simulink model "a1_walking"  (R2022b)
settings: Solver=VariableStepAuto  StartTime=0.0  StopTime=0.2  RelTol=1e-3
values from neighbouring files (symbols this model uses):
  m = 12    [MPC_Controller.m]    (also in QP_Controller.m; TASK1_rotating_mpc.m; TASK1_walking_backward_mpc.m; TASK1_walking_forward_mpc.m)
  N = 10    [MPC_Controller.m]
undefined symbols (not defined in the file or in its folder): X, Y, Z
libraries: sm_lib x188, nesl_utility x113
(part 2 of 5)

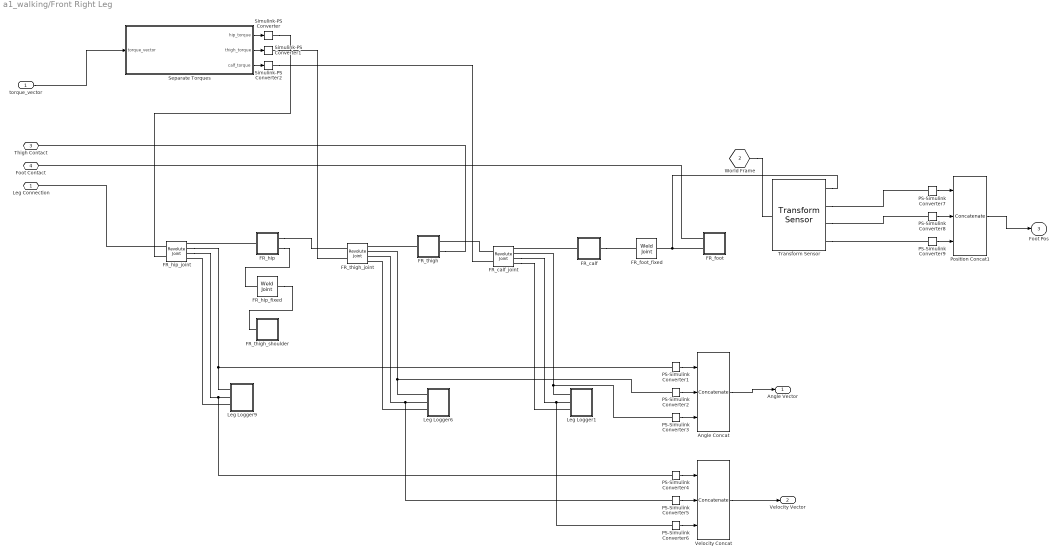
== system a1_walking/Front Right Leg ==
  torque_vector : Inport
  Angle Concat : Concatenate  NumInputs=3
  FR_calf : Subsystem
  FR_calf_joint : sm_lib/Joints/Revolute Joint  JointMode=Normal  SenseConstraintForce=off  SenseConstraintForceX=off  SenseConstraintForceY=off  SenseConstraintForceZ=off  SenseConstraintTorque=off  SenseConstraintTorqueX=off  SenseConstraintTorqueY=off  SenseConstraintTorqueZ=off  SenseTotalForce=off  SenseTotalForceX=off  SenseTotalForceY=off  SenseTotalForceZ=off  SenseTotalTorque=off  SenseTotalTorqueX=off  SenseTotalTorqueY=off  SenseTotalTorqueZ=off  CompositeWrenchDir=FollowerOnBase  CompositeWrenchFrame=BaseFrame  EquilibriumPosition=0  EquilibriumPositionUnits=deg  SpringStiffness=0  SpringStiffnessUnits=N*m/deg  DampingCoefficient=0.01  DampingCoefficientUnits=kg*m^2/(rad*s)  TorqueActuationMode=InputTorque  MotionActuationMode=ComputedMotion  SensePosition=on  SenseVelocity=on  SenseAcceleration=off  SenseTorqueForce=on  SenseLowerLimitTorqueForce=off  SenseUpperLimitTorqueForce=off  LowerLimitSpecify=on  LowerLimitBound=-2.69653369433  LowerLimitBoundUnits=rad  LowerLimitStiffness=1e4  LowerLimitStiffnessUnits=N*m/deg  LowerLimitDamping=10  LowerLimitDampingUnits=N*m/(deg/s)  LowerLimitTransitionRegionWidth=0.1  LowerLimitTransitionRegionWidthUnits=deg  UpperLimitSpecify=on  UpperLimitBound=-0.916297857297  UpperLimitBoundUnits=rad  UpperLimitStiffness=1e4  UpperLimitStiffnessUnits=N*m/deg  UpperLimitDamping=10  UpperLimitDampingUnits=N*m/(deg/s)  UpperLimitTransitionRegionWidth=0.1  UpperLimitTransitionRegionWidthUnits=deg  PositionTargetSpecify=on  PositionTargetPriority=High  PositionTargetValue=-2.5  PositionTargetValueUnits=rad  VelocityTargetSpecify=on  VelocityTargetPriority=High  VelocityTargetValue=0  VelocityTargetValueUnits=rad/s
  FR_foot : Subsystem
  FR_foot_fixed : sm_lib/Joints/Weld Joint  JointMode=Normal  SenseConstraintForce=off  SenseConstraintForceX=off  SenseConstraintForceY=off  SenseConstraintForceZ=off  SenseConstraintTorque=off  SenseConstraintTorqueX=off  SenseConstraintTorqueY=off  SenseConstraintTorqueZ=off  SenseTotalForce=off  SenseTotalForceX=off  SenseTotalForceY=off  SenseTotalForceZ=off  SenseTotalTorque=off  SenseTotalTorqueX=off  SenseTotalTorqueY=off  SenseTotalTorqueZ=off  CompositeWrenchDir=FollowerOnBase  CompositeWrenchFrame=BaseFrame
  FR_hip : Subsystem
  FR_hip_fixed : sm_lib/Joints/Weld Joint  JointMode=Normal  SenseConstraintForce=off  SenseConstraintForceX=off  SenseConstraintForceY=off  SenseConstraintForceZ=off  SenseConstraintTorque=off  SenseConstraintTorqueX=off  SenseConstraintTorqueY=off  SenseConstraintTorqueZ=off  SenseTotalForce=off  SenseTotalForceX=off  SenseTotalForceY=off  SenseTotalForceZ=off  SenseTotalTorque=off  SenseTotalTorqueX=off  SenseTotalTorqueY=off  SenseTotalTorqueZ=off  CompositeWrenchDir=FollowerOnBase  CompositeWrenchFrame=BaseFrame
  FR_hip_joint : sm_lib/Joints/Revolute Joint  JointMode=Normal  SenseConstraintForce=off  SenseConstraintForceX=off  SenseConstraintForceY=off  SenseConstraintForceZ=off  SenseConstraintTorque=off  SenseConstraintTorqueX=off  SenseConstraintTorqueY=off  SenseConstraintTorqueZ=off  SenseTotalForce=off  SenseTotalForceX=off  SenseTotalForceY=off  SenseTotalForceZ=off  SenseTotalTorque=off  SenseTotalTorqueX=off  SenseTotalTorqueY=off  SenseTotalTorqueZ=off  CompositeWrenchDir=FollowerOnBase  CompositeWrenchFrame=BaseFrame  EquilibriumPosition=0  EquilibriumPositionUnits=deg  SpringStiffness=0  SpringStiffnessUnits=N*m/deg  DampingCoefficient=0.01  DampingCoefficientUnits=kg*m^2/(rad*s)  TorqueActuationMode=InputTorque  MotionActuationMode=ComputedMotion  SensePosition=on  SenseVelocity=on  SenseAcceleration=off  SenseTorqueForce=on  SenseLowerLimitTorqueForce=off  SenseUpperLimitTorqueForce=off  LowerLimitSpecify=on  LowerLimitBound=-0.802851455917  LowerLimitBoundUnits=rad  LowerLimitStiffness=1e4  LowerLimitStiffnessUnits=N*m/deg  LowerLimitDamping=10  LowerLimitDampingUnits=N*m/(deg/s)  LowerLimitTransitionRegionWidth=0.1  LowerLimitTransitionRegionWidthUnits=deg  UpperLimitSpecify=on  UpperLimitBound=0.802851455917  UpperLimitBoundUnits=rad  UpperLimitStiffness=1e4  UpperLimitStiffnessUnits=N*m/deg  UpperLimitDamping=10  UpperLimitDampingUnits=N*m/(deg/s)  UpperLimitTransitionRegionWidth=0.1  UpperLimitTransitionRegionWidthUnits=deg  PositionTargetSpecify=on  PositionTargetPriority=High  PositionTargetValue=0  PositionTargetValueUnits=rad  VelocityTargetSpecify=on  VelocityTargetPriority=High  VelocityTargetValue=0  VelocityTargetValueUnits=deg/s
  FR_thigh : Subsystem
  FR_thigh_joint : sm_lib/Joints/Revolute Joint  JointMode=Normal  SenseConstraintForce=off  SenseConstraintForceX=off  SenseConstraintForceY=off  SenseConstraintForceZ=off  SenseConstraintTorque=off  SenseConstraintTorqueX=off  SenseConstraintTorqueY=off  SenseConstraintTorqueZ=off  SenseTotalForce=off  SenseTotalForceX=off  SenseTotalForceY=off  SenseTotalForceZ=off  SenseTotalTorque=off  SenseTotalTorqueX=off  SenseTotalTorqueY=off  SenseTotalTorqueZ=off  CompositeWrenchDir=FollowerOnBase  CompositeWrenchFrame=BaseFrame  EquilibriumPosition=0  EquilibriumPositionUnits=deg  SpringStiffness=0  SpringStiffnessUnits=N*m/deg  DampingCoefficient=0.01  DampingCoefficientUnits=kg*m^2/(rad*s)  TorqueActuationMode=InputTorque  MotionActuationMode=ComputedMotion  SensePosition=on  SenseVelocity=on  SenseAcceleration=off  SenseTorqueForce=on  SenseLowerLimitTorqueForce=off  SenseUpperLimitTorqueForce=off  LowerLimitSpecify=on  LowerLimitBound=-1.0471975512  LowerLimitBoundUnits=rad  LowerLimitStiffness=1e4  LowerLimitStiffnessUnits=N*m/deg  LowerLimitDamping=10  LowerLimitDampingUnits=N*m/(deg/s)  LowerLimitTransitionRegionWidth=0.1  LowerLimitTransitionRegionWidthUnits=deg  UpperLimitSpecify=on  UpperLimitBound=4.18879020479  UpperLimitBoundUnits=rad  UpperLimitStiffness=1e4  UpperLimitStiffnessUnits=N*m/deg  UpperLimitDamping=10  UpperLimitDampingUnits=N*m/(deg/s)  UpperLimitTransitionRegionWidth=0.1  UpperLimitTransitionRegionWidthUnits=deg  PositionTargetSpecify=on  PositionTargetPriority=High  PositionTargetValue=1  PositionTargetValueUnits=rad  VelocityTargetSpecify=on  VelocityTargetPriority=High  VelocityTargetValue=0  VelocityTargetValueUnits=deg/s
  FR_thigh_shoulder : Subsystem
  Leg Logger1 : Subsystem
  Leg Logger6 : Subsystem
  Leg Logger9 : Subsystem
  PS-Simulink Converter{1..9} (9 alike) : nesl_utility/PS-Simulink Converter  PhysicalDomain=network_engine_domain  SubClassName=ps_output  LeftPortType=input  RightPortType=output  PseudoPeriodic=off  Frequencies=[]  VectorFormat=inherit  Unit=inherit  AffineConversion=off
  Position Concat1 : Concatenate  NumInputs=3
  Separate Torques : MATLAB Function  TreatAsAtomicUnit=on
  Simulink-PS Converter : nesl_utility/Simulink-PS Converter  PhysicalDomain=network_engine_domain  SubClassName=ps_input  LeftPortType=input  RightPortType=output  PseudoPeriodic=off  Frequencies=[]  NoiseDistribution=none  NoiseParameters=[]  Unit=1  AffineConversion=off  FilteringAndDerivatives=provide  SimscapeFilterOrder=1  InputFilterTimeConstant=0.001  UdotUserProvided=0
  Simulink-PS Converter1 : nesl_utility/Simulink-PS Converter  PhysicalDomain=network_engine_domain  SubClassName=ps_input  LeftPortType=input  RightPortType=output  PseudoPeriodic=off  Frequencies=[]  NoiseDistribution=none  NoiseParameters=[]  Unit=1  AffineConversion=off  FilteringAndDerivatives=provide  SimscapeFilterOrder=1  InputFilterTimeConstant=0.001  UdotUserProvided=0
  Simulink-PS Converter2 : nesl_utility/Simulink-PS Converter  PhysicalDomain=network_engine_domain  SubClassName=ps_input  LeftPortType=input  RightPortType=output  PseudoPeriodic=off  Frequencies=[]  NoiseDistribution=none  NoiseParameters=[]  Unit=1  AffineConversion=off  FilteringAndDerivatives=provide  SimscapeFilterOrder=1  InputFilterTimeConstant=0.001  UdotUserProvided=0
  Transform Sensor : sm_lib/Frames and Transforms/Transform Sensor  MeasurementFrame=World  SenseAngle=off  SenseAxis=off  SenseQ=off  SenseR=off  SenseRotationSequence=off  RotationSequence=XYX  SenseOmegaX=off  SenseOmegaY=off  SenseOmegaZ=off  SenseQDot=off  SenseRDot=off  SenseAlphaX=off  SenseAlphaY=off  SenseAlphaZ=off  SenseQDDot=off  SenseRDDot=off  SenseX=on  SenseY=on  SenseZ=on  SenseRad=off  SenseAzim=off  SenseDist=off  SenseInc=off  SenseXDot=off  SenseYDot=off  SenseZDot=off  SenseRadDot=off  SenseAzimDot=off  SenseDistDot=off  SenseIncDot=off  SenseXDDot=off  SenseYDDot=off  SenseZDDot=off  SenseRadDDot=off  SenseAzimDDot=off  SenseDistDDot=off  SenseIncDDot=off
  Velocity Concat : Concatenate  NumInputs=3
  Leg Connection : PMIOPort  Side=Left
  World Frame : PMIOPort  Port=2  Side=Left
  Thigh Contact : PMIOPort  Port=3  Side=Left
  Foot Contact : PMIOPort  Port=4  Side=Left
  Angle Vector : Outport
  Velocity Vector : Outport  Port=2
  Foot Pos : Outport  Port=3
  wires:
  Separate Torques/2(thigh_torque) -> Simulink-PS Converter1/1
  Separate Torques/1(hip_torque) -> Simulink-PS Converter/1
  Separate Torques/3(calf_torque) -> Simulink-PS Converter2/1
  Velocity Concat/1 -> Velocity Vector/1
  PS-Simulink Converter4/1 -> Velocity Concat/1
  PS-Simulink Converter3/1 -> Angle Concat/3
  PS-Simulink Converter1/1 -> Angle Concat/1
  PS-Simulink Converter6/1 -> Velocity Concat/3
  PS-Simulink Converter5/1 -> Velocity Concat/2
  PS-Simulink Converter2/1 -> Angle Concat/2
  torque_vector/1 -> Separate Torques/1(torque_vector)
  Angle Concat/1 -> Angle Vector/1
  PS-Simulink Converter9/1 -> Position Concat1/3
  PS-Simulink Converter8/1 -> Position Concat1/2
  PS-Simulink Converter7/1 -> Position Concat1/1
  Position Concat1/1 -> Foot Pos/1
  connections:
  FR_calf_joint/RConn3 -- PS-Simulink Converter6/LConn1 -- Leg Logger1/LConn2
  Leg Logger6/LConn2 -- PS-Simulink Converter5/LConn1 -- FR_thigh_joint/RConn3
  Leg Logger6/LConn1 -- FR_thigh_joint/RConn2 -- PS-Simulink Converter2/LConn1
  FR_calf_joint/RConn4 -- Leg Logger1/LConn3
  FR_hip/RConn1 -- FR_thigh_joint/LConn1
  FR_thigh/LConn1 -- FR_thigh_joint/RConn1
  FR_hip_joint/RConn2 -- PS-Simulink Converter1/LConn1 -- Leg Logger9/LConn1
  Leg Logger9/LConn3 -- FR_hip_joint/RConn4
  FR_hip_fixed/RConn1 -- FR_thigh_shoulder/LConn1
  FR_calf_joint/LConn1 -- FR_thigh/RConn1
  Leg Logger6/LConn3 -- FR_thigh_joint/RConn4
  FR_hip/RConn2 -- FR_hip_fixed/LConn1
  FR_hip_joint/RConn3 -- PS-Simulink Converter4/LConn1 -- Leg Logger9/LConn2
  FR_thigh/RConn2 -- Thigh Contact/RConn1
  FR_hip_joint/LConn1 -- Leg Connection/RConn1
  Leg Logger1/LConn1 -- PS-Simulink Converter3/LConn1 -- FR_calf_joint/RConn2
  FR_calf/LConn1 -- FR_calf_joint/RConn1
  FR_calf/RConn1 -- FR_foot_fixed/LConn1
  FR_hip/LConn1 -- FR_hip_joint/RConn1
  FR_foot/LConn1 -- Foot Contact/RConn1
  FR_foot/LConn2 -- Transform Sensor/RConn1 -- FR_foot_fixed/RConn1
  Simulink-PS Converter1/RConn1 -- FR_thigh_joint/LConn2
  Simulink-PS Converter/RConn1 -- FR_hip_joint/LConn2
  Simulink-PS Converter2/RConn1 -- FR_calf_joint/LConn2
  Transform Sensor/RConn2 -- PS-Simulink Converter7/LConn1
  Transform Sensor/RConn3 -- PS-Simulink Converter8/LConn1
  Transform Sensor/RConn4 -- PS-Simulink Converter9/LConn1
  World Frame/RConn1 -- Transform Sensor/LConn1

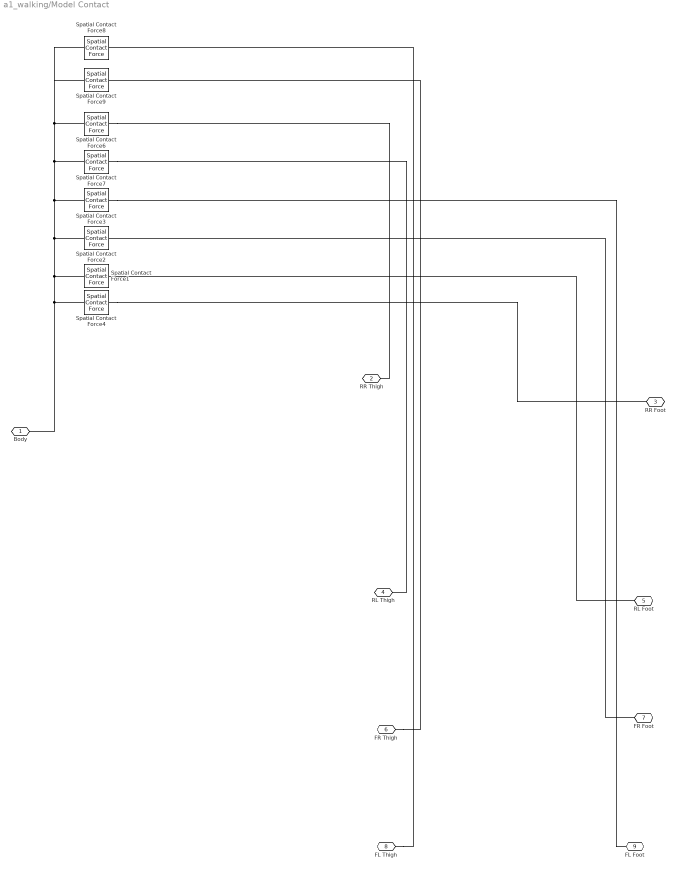
== system a1_walking/Model Contact ==
  Spatial Contact Force{1..4,6..9} (8 alike) : sm_lib/Forces and Torques/Spatial Contact Force  SenseContactBaseRotation=off  SenseContactBaseTranslation=off  CoefficientOfDynamicFriction=0.3  CoefficientOfStaticFriction=0.5  NormalDamping=1e3  NormalDampingUnits=N/(m/s)  SenseContactSignal=off  NormalStiffness=1e6  NormalStiffnessUnits=N/m  FrictionalCriticalVelocity=1e-3  FrictionalCriticalVelocityUnits=m/s  ZeroCrossDetectContactStartAndEnd=off  SenseContactFollowerRotation=off  SenseContactFollowerTranslation=off  FrictionType=SmoothStickSlip  SenseFrictionalForceMagnitude=off  SenseNormalForceMagnitude=off  NormalForceType=SmoothSpringDamper  SenseNormalVelocity=off  SenseSeparationDistance=off  SenseTangentialVelocity=off  NormalTransitionRegionWidth=1e-4  NormalTransitionRegionWidthUnits=m
  Body : PMIOPort  Side=Left
  RR Thigh : PMIOPort  Port=2  Side=Right
  RR Foot : PMIOPort  Port=3  Side=Right
  RL Thigh : PMIOPort  Port=4  Side=Right
  RL Foot : PMIOPort  Port=5  Side=Right
  FR Thigh : PMIOPort  Port=6  Side=Right
  FR Foot : PMIOPort  Port=7  Side=Right
  FL Thigh : PMIOPort  Port=8  Side=Right
  FL Foot : PMIOPort  Port=9  Side=Right
  connections:
  Spatial Contact Force3/RConn1 -- FL Foot/RConn1
  FL Thigh/RConn1 -- Spatial Contact Force8/RConn1
  Spatial Contact Force7/RConn1 -- RL Thigh/RConn1
  RL Foot/RConn1 -- Spatial Contact Force1/RConn1
  FR Thigh/RConn1 -- Spatial Contact Force9/RConn1
  Spatial Contact Force4/LConn1 -- Body/RConn1 -- Spatial Contact Force7/LConn1 -- Spatial Contact Force6/LConn1 -- Spatial Contact Force9/LConn1 -- Spatial Contact Force8/LConn1 -- Spatial Contact Force3/LConn1 -- Spatial Contact Force2/LConn1 -- Spatial Contact Force1/LConn1
  FR Foot/RConn1 -- Spatial Contact Force2/RConn1
  Spatial Contact Force6/RConn1 -- RR Thigh/RConn1
  Spatial Contact Force4/RConn1 -- RR Foot/RConn1

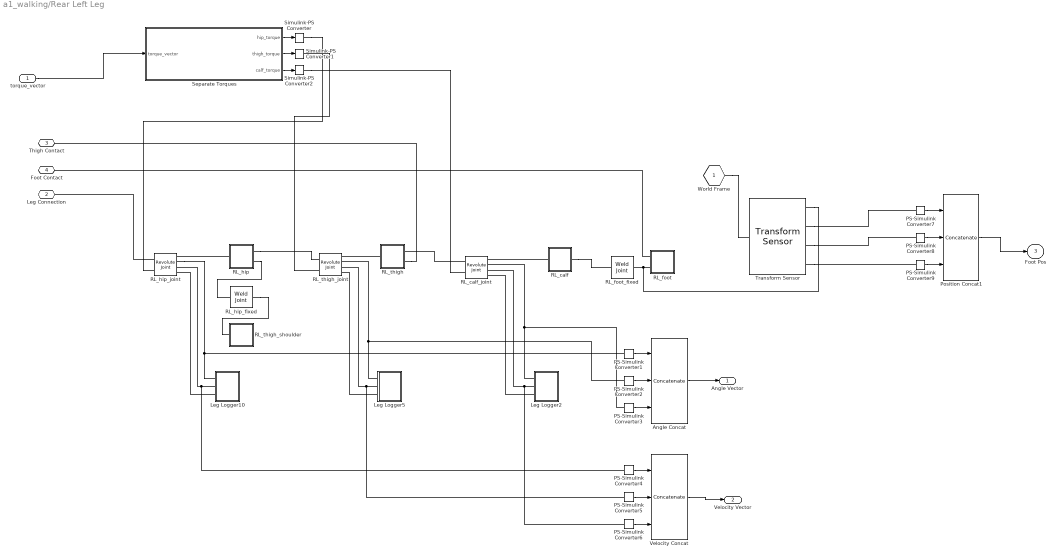
== system a1_walking/Rear Left Leg ==
  torque_vector : Inport
  Angle Concat : Concatenate  NumInputs=3
  Leg Logger10 : Subsystem
  Leg Logger2 : Subsystem
  Leg Logger5 : Subsystem
  PS-Simulink Converter{1..9} (9 alike) : nesl_utility/PS-Simulink Converter  PhysicalDomain=network_engine_domain  SubClassName=ps_output  LeftPortType=input  RightPortType=output  PseudoPeriodic=off  Frequencies=[]  VectorFormat=inherit  Unit=inherit  AffineConversion=off
  Position Concat1 : Concatenate  NumInputs=3
  RL_calf : Subsystem
  RL_calf_joint : sm_lib/Joints/Revolute Joint  JointMode=Normal  SenseConstraintForce=off  SenseConstraintForceX=off  SenseConstraintForceY=off  SenseConstraintForceZ=off  SenseConstraintTorque=off  SenseConstraintTorqueX=off  SenseConstraintTorqueY=off  SenseConstraintTorqueZ=off  SenseTotalForce=off  SenseTotalForceX=off  SenseTotalForceY=off  SenseTotalForceZ=off  SenseTotalTorque=off  SenseTotalTorqueX=off  SenseTotalTorqueY=off  SenseTotalTorqueZ=off  CompositeWrenchDir=FollowerOnBase  CompositeWrenchFrame=BaseFrame  EquilibriumPosition=0  EquilibriumPositionUnits=deg  SpringStiffness=0  SpringStiffnessUnits=N*m/deg  DampingCoefficient=0.01  DampingCoefficientUnits=kg*m^2/(rad*s)  TorqueActuationMode=InputTorque  MotionActuationMode=ComputedMotion  SensePosition=on  SenseVelocity=on  SenseAcceleration=off  SenseTorqueForce=on  SenseLowerLimitTorqueForce=off  SenseUpperLimitTorqueForce=off  LowerLimitSpecify=on  LowerLimitBound=-2.69653369433  LowerLimitBoundUnits=rad  LowerLimitStiffness=1e4  LowerLimitStiffnessUnits=N*m/deg  LowerLimitDamping=10  LowerLimitDampingUnits=N*m/(deg/s)  LowerLimitTransitionRegionWidth=0.1  LowerLimitTransitionRegionWidthUnits=deg  UpperLimitSpecify=on  UpperLimitBound=-0.916297857297  UpperLimitBoundUnits=rad  UpperLimitStiffness=1e4  UpperLimitStiffnessUnits=N*m/deg  UpperLimitDamping=10  UpperLimitDampingUnits=N*m/(deg/s)  UpperLimitTransitionRegionWidth=0.1  UpperLimitTransitionRegionWidthUnits=deg  PositionTargetSpecify=on  PositionTargetPriority=High  PositionTargetValue=-2.5  PositionTargetValueUnits=rad  VelocityTargetSpecify=on  VelocityTargetPriority=High  VelocityTargetValue=0  VelocityTargetValueUnits=deg/s
  RL_foot : Subsystem
  RL_foot_fixed : sm_lib/Joints/Weld Joint  JointMode=Normal  SenseConstraintForce=off  SenseConstraintForceX=off  SenseConstraintForceY=off  SenseConstraintForceZ=off  SenseConstraintTorque=off  SenseConstraintTorqueX=off  SenseConstraintTorqueY=off  SenseConstraintTorqueZ=off  SenseTotalForce=off  SenseTotalForceX=off  SenseTotalForceY=off  SenseTotalForceZ=off  SenseTotalTorque=off  SenseTotalTorqueX=off  SenseTotalTorqueY=off  SenseTotalTorqueZ=off  CompositeWrenchDir=FollowerOnBase  CompositeWrenchFrame=BaseFrame
  RL_hip : Subsystem
  RL_hip_fixed : sm_lib/Joints/Weld Joint  JointMode=Normal  SenseConstraintForce=off  SenseConstraintForceX=off  SenseConstraintForceY=off  SenseConstraintForceZ=off  SenseConstraintTorque=off  SenseConstraintTorqueX=off  SenseConstraintTorqueY=off  SenseConstraintTorqueZ=off  SenseTotalForce=off  SenseTotalForceX=off  SenseTotalForceY=off  SenseTotalForceZ=off  SenseTotalTorque=off  SenseTotalTorqueX=off  SenseTotalTorqueY=off  SenseTotalTorqueZ=off  CompositeWrenchDir=FollowerOnBase  CompositeWrenchFrame=BaseFrame
  RL_hip_joint : sm_lib/Joints/Revolute Joint  JointMode=Normal  SenseConstraintForce=off  SenseConstraintForceX=off  SenseConstraintForceY=off  SenseConstraintForceZ=off  SenseConstraintTorque=off  SenseConstraintTorqueX=off  SenseConstraintTorqueY=off  SenseConstraintTorqueZ=off  SenseTotalForce=off  SenseTotalForceX=off  SenseTotalForceY=off  SenseTotalForceZ=off  SenseTotalTorque=off  SenseTotalTorqueX=off  SenseTotalTorqueY=off  SenseTotalTorqueZ=off  CompositeWrenchDir=FollowerOnBase  CompositeWrenchFrame=BaseFrame  EquilibriumPosition=0  EquilibriumPositionUnits=deg  SpringStiffness=0  SpringStiffnessUnits=N*m/deg  DampingCoefficient=0.01  DampingCoefficientUnits=kg*m^2/(rad*s)  TorqueActuationMode=InputTorque  MotionActuationMode=ComputedMotion  SensePosition=on  SenseVelocity=on  SenseAcceleration=off  SenseTorqueForce=on  SenseLowerLimitTorqueForce=off  SenseUpperLimitTorqueForce=off  LowerLimitSpecify=on  LowerLimitBound=-0.802851455917  LowerLimitBoundUnits=rad  LowerLimitStiffness=1e4  LowerLimitStiffnessUnits=N*m/deg  LowerLimitDamping=10  LowerLimitDampingUnits=N*m/(deg/s)  LowerLimitTransitionRegionWidth=0.1  LowerLimitTransitionRegionWidthUnits=deg  UpperLimitSpecify=on  UpperLimitBound=0.802851455917  UpperLimitBoundUnits=rad  UpperLimitStiffness=1e4  UpperLimitStiffnessUnits=N*m/deg  UpperLimitDamping=10  UpperLimitDampingUnits=N*m/(deg/s)  UpperLimitTransitionRegionWidth=0.1  UpperLimitTransitionRegionWidthUnits=deg  PositionTargetSpecify=on  PositionTargetPriority=High  PositionTargetValue=0  PositionTargetValueUnits=rad  VelocityTargetSpecify=on  VelocityTargetPriority=High  VelocityTargetValue=0  VelocityTargetValueUnits=deg/s
  RL_thigh : Subsystem
  RL_thigh_joint : sm_lib/Joints/Revolute Joint  JointMode=Normal  SenseConstraintForce=off  SenseConstraintForceX=off  SenseConstraintForceY=off  SenseConstraintForceZ=off  SenseConstraintTorque=off  SenseConstraintTorqueX=off  SenseConstraintTorqueY=off  SenseConstraintTorqueZ=off  SenseTotalForce=off  SenseTotalForceX=off  SenseTotalForceY=off  SenseTotalForceZ=off  SenseTotalTorque=off  SenseTotalTorqueX=off  SenseTotalTorqueY=off  SenseTotalTorqueZ=off  CompositeWrenchDir=FollowerOnBase  CompositeWrenchFrame=BaseFrame  EquilibriumPosition=0  EquilibriumPositionUnits=deg  SpringStiffness=0  SpringStiffnessUnits=N*m/deg  DampingCoefficient=0.01  DampingCoefficientUnits=kg*m^2/(rad*s)  TorqueActuationMode=InputTorque  MotionActuationMode=ComputedMotion  SensePosition=on  SenseVelocity=on  SenseAcceleration=off  SenseTorqueForce=on  SenseLowerLimitTorqueForce=off  SenseUpperLimitTorqueForce=off  LowerLimitSpecify=on  LowerLimitBound=-1.0471975512  LowerLimitBoundUnits=rad  LowerLimitStiffness=1e4  LowerLimitStiffnessUnits=N*m/deg  LowerLimitDamping=10  LowerLimitDampingUnits=N*m/(deg/s)  LowerLimitTransitionRegionWidth=0.1  LowerLimitTransitionRegionWidthUnits=deg  UpperLimitSpecify=on  UpperLimitBound=4.18879020479  UpperLimitBoundUnits=rad  UpperLimitStiffness=1e4  UpperLimitStiffnessUnits=N*m/deg  UpperLimitDamping=10  UpperLimitDampingUnits=N*m/(deg/s)  UpperLimitTransitionRegionWidth=0.1  UpperLimitTransitionRegionWidthUnits=deg  PositionTargetSpecify=on  PositionTargetPriority=High  PositionTargetValue=1  PositionTargetValueUnits=rad  VelocityTargetSpecify=on  VelocityTargetPriority=High  VelocityTargetValue=0  VelocityTargetValueUnits=deg/s
  RL_thigh_shoulder : Subsystem
  Separate Torques : MATLAB Function  TreatAsAtomicUnit=on
  Simulink-PS Converter : nesl_utility/Simulink-PS Converter  PhysicalDomain=network_engine_domain  SubClassName=ps_input  LeftPortType=input  RightPortType=output  PseudoPeriodic=off  Frequencies=[]  NoiseDistribution=none  NoiseParameters=[]  Unit=1  AffineConversion=off  FilteringAndDerivatives=provide  SimscapeFilterOrder=1  InputFilterTimeConstant=0.001  UdotUserProvided=0
  Simulink-PS Converter1 : nesl_utility/Simulink-PS Converter  PhysicalDomain=network_engine_domain  SubClassName=ps_input  LeftPortType=input  RightPortType=output  PseudoPeriodic=off  Frequencies=[]  NoiseDistribution=none  NoiseParameters=[]  Unit=1  AffineConversion=off  FilteringAndDerivatives=provide  SimscapeFilterOrder=1  InputFilterTimeConstant=0.001  UdotUserProvided=0
  Simulink-PS Converter2 : nesl_utility/Simulink-PS Converter  PhysicalDomain=network_engine_domain  SubClassName=ps_input  LeftPortType=input  RightPortType=output  PseudoPeriodic=off  Frequencies=[]  NoiseDistribution=none  NoiseParameters=[]  Unit=1  AffineConversion=off  FilteringAndDerivatives=provide  SimscapeFilterOrder=1  InputFilterTimeConstant=0.001  UdotUserProvided=0
  Transform Sensor : sm_lib/Frames and Transforms/Transform Sensor  MeasurementFrame=World  SenseAngle=off  SenseAxis=off  SenseQ=off  SenseR=off  SenseRotationSequence=off  RotationSequence=XYX  SenseOmegaX=off  SenseOmegaY=off  SenseOmegaZ=off  SenseQDot=off  SenseRDot=off  SenseAlphaX=off  SenseAlphaY=off  SenseAlphaZ=off  SenseQDDot=off  SenseRDDot=off  SenseX=on  SenseY=on  SenseZ=on  SenseRad=off  SenseAzim=off  SenseDist=off  SenseInc=off  SenseXDot=off  SenseYDot=off  SenseZDot=off  SenseRadDot=off  SenseAzimDot=off  SenseDistDot=off  SenseIncDot=off  SenseXDDot=off  SenseYDDot=off  SenseZDDot=off  SenseRadDDot=off  SenseAzimDDot=off  SenseDistDDot=off  SenseIncDDot=off
  Velocity Concat : Concatenate  NumInputs=3
  World Frame : PMIOPort  Side=Left
  Leg Connection : PMIOPort  Port=2  Side=Left
  Thigh Contact : PMIOPort  Port=3  Side=Left
  Foot Contact : PMIOPort  Port=4  Side=Left
  Angle Vector : Outport
  Velocity Vector : Outport  Port=2
  Foot Pos : Outport  Port=3
  wires:
  Separate Torques/1(hip_torque) -> Simulink-PS Converter/1
  Separate Torques/2(thigh_torque) -> Simulink-PS Converter1/1
  Separate Torques/3(calf_torque) -> Simulink-PS Converter2/1
  PS-Simulink Converter1/1 -> Angle Concat/1
  PS-Simulink Converter3/1 -> Angle Concat/3
  PS-Simulink Converter2/1 -> Angle Concat/2
  PS-Simulink Converter4/1 -> Velocity Concat/1
  PS-Simulink Converter5/1 -> Velocity Concat/2
  PS-Simulink Converter6/1 -> Velocity Concat/3
  torque_vector/1 -> Separate Torques/1(torque_vector)
  Angle Concat/1 -> Angle Vector/1
  Velocity Concat/1 -> Velocity Vector/1
  PS-Simulink Converter8/1 -> Position Concat1/2
  PS-Simulink Converter9/1 -> Position Concat1/3
  PS-Simulink Converter7/1 -> Position Concat1/1
  Position Concat1/1 -> Foot Pos/1
  connections:
  RL_thigh/RConn2 -- Thigh Contact/RConn1
  RL_foot/LConn2 -- Transform Sensor/RConn1 -- RL_foot_fixed/RConn1
  RL_hip/RConn1 -- RL_thigh_joint/LConn1
  RL_hip_fixed/RConn1 -- RL_thigh_shoulder/LConn1
  Leg Logger5/LConn2 -- PS-Simulink Converter5/LConn1 -- RL_thigh_joint/RConn3
  Leg Logger10/LConn2 -- PS-Simulink Converter4/LConn1 -- RL_hip_joint/RConn3
  Leg Logger10/LConn3 -- RL_hip_joint/RConn4
  Leg Logger2/LConn3 -- RL_calf_joint/RConn4
  RL_hip/RConn2 -- RL_hip_fixed/LConn1
  RL_hip/LConn1 -- RL_hip_joint/RConn1
  RL_calf/RConn1 -- RL_foot_fixed/LConn1
  Leg Logger5/LConn1 -- PS-Simulink Converter2/LConn1 -- RL_thigh_joint/RConn2
  RL_thigh/LConn1 -- RL_thigh_joint/RConn1
  RL_hip_joint/RConn2 -- PS-Simulink Converter1/LConn1 -- Leg Logger10/LConn1
  Leg Logger2/LConn1 -- PS-Simulink Converter3/LConn1 -- RL_calf_joint/RConn2
  RL_hip_joint/LConn1 -- Leg Connection/RConn1
  RL_calf/LConn1 -- RL_calf_joint/RConn1
  RL_calf_joint/LConn1 -- RL_thigh/RConn1
  Leg Logger2/LConn2 -- PS-Simulink Converter6/LConn1 -- RL_calf_joint/RConn3
  RL_foot/LConn1 -- Foot Contact/RConn1
  Leg Logger5/LConn3 -- RL_thigh_joint/RConn4
  Simulink-PS Converter/RConn1 -- RL_hip_joint/LConn2
  Simulink-PS Converter1/RConn1 -- RL_thigh_joint/LConn2
  Simulink-PS Converter2/RConn1 -- RL_calf_joint/LConn2
  World Frame/RConn1 -- Transform Sensor/LConn1
  Transform Sensor/RConn2 -- PS-Simulink Converter7/LConn1
  Transform Sensor/RConn3 -- PS-Simulink Converter8/LConn1
  Transform Sensor/RConn4 -- PS-Simulink Converter9/LConn1

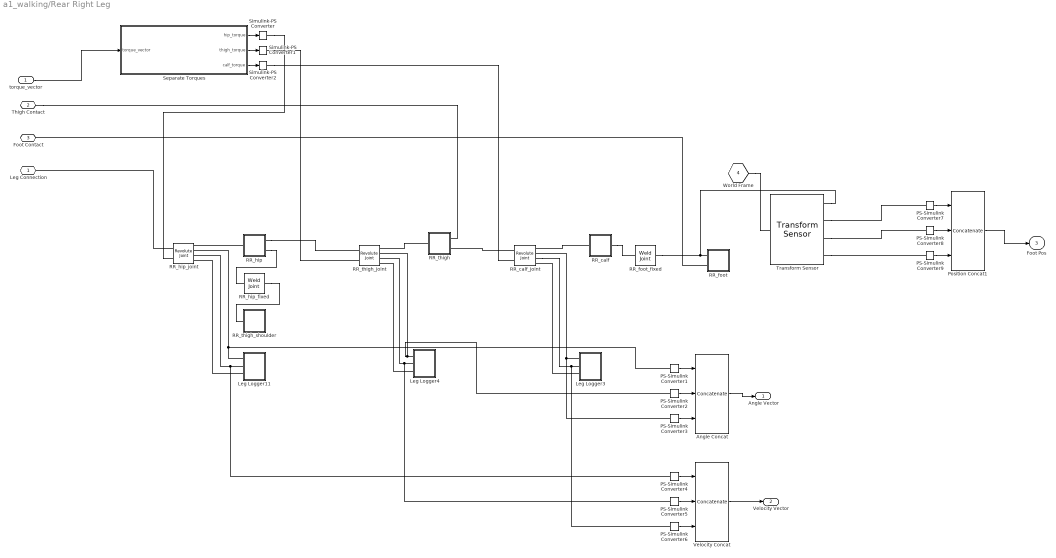
== system a1_walking/Rear Right Leg ==
  torque_vector : Inport
  Angle Concat : Concatenate  NumInputs=3
  Leg Logger11 : Subsystem
  Leg Logger3 : Subsystem
  Leg Logger4 : Subsystem
  PS-Simulink Converter{1..9} (9 alike) : nesl_utility/PS-Simulink Converter  PhysicalDomain=network_engine_domain  SubClassName=ps_output  LeftPortType=input  RightPortType=output  PseudoPeriodic=off  Frequencies=[]  VectorFormat=inherit  Unit=inherit  AffineConversion=off
  Position Concat1 : Concatenate  NumInputs=3
  RR_calf : Subsystem
  RR_calf_joint : sm_lib/Joints/Revolute Joint  JointMode=Normal  SenseConstraintForce=off  SenseConstraintForceX=off  SenseConstraintForceY=off  SenseConstraintForceZ=off  SenseConstraintTorque=off  SenseConstraintTorqueX=off  SenseConstraintTorqueY=off  SenseConstraintTorqueZ=off  SenseTotalForce=off  SenseTotalForceX=off  SenseTotalForceY=off  SenseTotalForceZ=off  SenseTotalTorque=off  SenseTotalTorqueX=off  SenseTotalTorqueY=off  SenseTotalTorqueZ=off  CompositeWrenchDir=FollowerOnBase  CompositeWrenchFrame=BaseFrame  EquilibriumPosition=0  EquilibriumPositionUnits=deg  SpringStiffness=0  SpringStiffnessUnits=N*m/deg  DampingCoefficient=0.01  DampingCoefficientUnits=kg*m^2/(rad*s)  TorqueActuationMode=InputTorque  MotionActuationMode=ComputedMotion  SensePosition=on  SenseVelocity=on  SenseAcceleration=off  SenseTorqueForce=on  SenseLowerLimitTorqueForce=off  SenseUpperLimitTorqueForce=off  LowerLimitSpecify=on  LowerLimitBound=-2.69653369433  LowerLimitBoundUnits=rad  LowerLimitStiffness=1e4  LowerLimitStiffnessUnits=N*m/deg  LowerLimitDamping=10  LowerLimitDampingUnits=N*m/(deg/s)  LowerLimitTransitionRegionWidth=0.1  LowerLimitTransitionRegionWidthUnits=deg  UpperLimitSpecify=on  UpperLimitBound=-0.916297857297  UpperLimitBoundUnits=rad  UpperLimitStiffness=1e4  UpperLimitStiffnessUnits=N*m/deg  UpperLimitDamping=10  UpperLimitDampingUnits=N*m/(deg/s)  UpperLimitTransitionRegionWidth=0.1  UpperLimitTransitionRegionWidthUnits=deg  PositionTargetSpecify=on  PositionTargetPriority=High  PositionTargetValue=-2.5  PositionTargetValueUnits=rad  VelocityTargetSpecify=on  VelocityTargetPriority=High  VelocityTargetValue=0  VelocityTargetValueUnits=deg/s
  RR_foot : Subsystem
  RR_foot_fixed : sm_lib/Joints/Weld Joint  JointMode=Normal  SenseConstraintForce=off  SenseConstraintForceX=off  SenseConstraintForceY=off  SenseConstraintForceZ=off  SenseConstraintTorque=off  SenseConstraintTorqueX=off  SenseConstraintTorqueY=off  SenseConstraintTorqueZ=off  SenseTotalForce=off  SenseTotalForceX=off  SenseTotalForceY=off  SenseTotalForceZ=off  SenseTotalTorque=off  SenseTotalTorqueX=off  SenseTotalTorqueY=off  SenseTotalTorqueZ=off  CompositeWrenchDir=FollowerOnBase  CompositeWrenchFrame=BaseFrame
  RR_hip : Subsystem
  RR_hip_fixed : sm_lib/Joints/Weld Joint  JointMode=Normal  SenseConstraintForce=off  SenseConstraintForceX=off  SenseConstraintForceY=off  SenseConstraintForceZ=off  SenseConstraintTorque=off  SenseConstraintTorqueX=off  SenseConstraintTorqueY=off  SenseConstraintTorqueZ=off  SenseTotalForce=off  SenseTotalForceX=off  SenseTotalForceY=off  SenseTotalForceZ=off  SenseTotalTorque=off  SenseTotalTorqueX=off  SenseTotalTorqueY=off  SenseTotalTorqueZ=off  CompositeWrenchDir=FollowerOnBase  CompositeWrenchFrame=BaseFrame
  RR_hip_joint : sm_lib/Joints/Revolute Joint  JointMode=Normal  SenseConstraintForce=off  SenseConstraintForceX=off  SenseConstraintForceY=off  SenseConstraintForceZ=off  SenseConstraintTorque=off  SenseConstraintTorqueX=off  SenseConstraintTorqueY=off  SenseConstraintTorqueZ=off  SenseTotalForce=off  SenseTotalForceX=off  SenseTotalForceY=off  SenseTotalForceZ=off  SenseTotalTorque=off  SenseTotalTorqueX=off  SenseTotalTorqueY=off  SenseTotalTorqueZ=off  CompositeWrenchDir=FollowerOnBase  CompositeWrenchFrame=BaseFrame  EquilibriumPosition=0  EquilibriumPositionUnits=deg  SpringStiffness=0  SpringStiffnessUnits=N*m/deg  DampingCoefficient=0.01  DampingCoefficientUnits=kg*m^2/(rad*s)  TorqueActuationMode=InputTorque  MotionActuationMode=ComputedMotion  SensePosition=on  SenseVelocity=on  SenseAcceleration=off  SenseTorqueForce=on  SenseLowerLimitTorqueForce=off  SenseUpperLimitTorqueForce=off  LowerLimitSpecify=on  LowerLimitBound=-0.802851455917  LowerLimitBoundUnits=rad  LowerLimitStiffness=1e4  LowerLimitStiffnessUnits=N*m/deg  LowerLimitDamping=10  LowerLimitDampingUnits=N*m/(deg/s)  LowerLimitTransitionRegionWidth=0.1  LowerLimitTransitionRegionWidthUnits=deg  UpperLimitSpecify=on  UpperLimitBound=0.802851455917  UpperLimitBoundUnits=rad  UpperLimitStiffness=1e4  UpperLimitStiffnessUnits=N*m/deg  UpperLimitDamping=10  UpperLimitDampingUnits=N*m/(deg/s)  UpperLimitTransitionRegionWidth=0.1  UpperLimitTransitionRegionWidthUnits=deg  PositionTargetSpecify=on  PositionTargetPriority=High  PositionTargetValue=0  PositionTargetValueUnits=rad  VelocityTargetSpecify=on  VelocityTargetPriority=High  VelocityTargetValue=0  VelocityTargetValueUnits=deg/s
  RR_thigh : Subsystem
  RR_thigh_joint : sm_lib/Joints/Revolute Joint  JointMode=Normal  SenseConstraintForce=off  SenseConstraintForceX=off  SenseConstraintForceY=off  SenseConstraintForceZ=off  SenseConstraintTorque=off  SenseConstraintTorqueX=off  SenseConstraintTorqueY=off  SenseConstraintTorqueZ=off  SenseTotalForce=off  SenseTotalForceX=off  SenseTotalForceY=off  SenseTotalForceZ=off  SenseTotalTorque=off  SenseTotalTorqueX=off  SenseTotalTorqueY=off  SenseTotalTorqueZ=off  CompositeWrenchDir=FollowerOnBase  CompositeWrenchFrame=BaseFrame  EquilibriumPosition=0  EquilibriumPositionUnits=deg  SpringStiffness=0  SpringStiffnessUnits=N*m/deg  DampingCoefficient=0.01  DampingCoefficientUnits=kg*m^2/(rad*s)  TorqueActuationMode=InputTorque  MotionActuationMode=ComputedMotion  SensePosition=on  SenseVelocity=on  SenseAcceleration=off  SenseTorqueForce=on  SenseLowerLimitTorqueForce=off  SenseUpperLimitTorqueForce=off  LowerLimitSpecify=on  LowerLimitBound=-1.0471975512  LowerLimitBoundUnits=rad  LowerLimitStiffness=1e4  LowerLimitStiffnessUnits=N*m/deg  LowerLimitDamping=10  LowerLimitDampingUnits=N*m/(deg/s)  LowerLimitTransitionRegionWidth=0.1  LowerLimitTransitionRegionWidthUnits=deg  UpperLimitSpecify=on  UpperLimitBound=4.18879020479  UpperLimitBoundUnits=rad  UpperLimitStiffness=1e4  UpperLimitStiffnessUnits=N*m/deg  UpperLimitDamping=10  UpperLimitDampingUnits=N*m/(deg/s)  UpperLimitTransitionRegionWidth=0.1  UpperLimitTransitionRegionWidthUnits=deg  PositionTargetSpecify=on  PositionTargetPriority=High  PositionTargetValue=1  PositionTargetValueUnits=rad  VelocityTargetSpecify=on  VelocityTargetPriority=High  VelocityTargetValue=0  VelocityTargetValueUnits=deg/s
  RR_thigh_shoulder : Subsystem
  Separate Torques : MATLAB Function  TreatAsAtomicUnit=on
  Simulink-PS Converter : nesl_utility/Simulink-PS Converter  PhysicalDomain=network_engine_domain  SubClassName=ps_input  LeftPortType=input  RightPortType=output  PseudoPeriodic=off  Frequencies=[]  NoiseDistribution=none  NoiseParameters=[]  Unit=1  AffineConversion=off  FilteringAndDerivatives=provide  SimscapeFilterOrder=1  InputFilterTimeConstant=0.001  UdotUserProvided=0
  Simulink-PS Converter1 : nesl_utility/Simulink-PS Converter  PhysicalDomain=network_engine_domain  SubClassName=ps_input  LeftPortType=input  RightPortType=output  PseudoPeriodic=off  Frequencies=[]  NoiseDistribution=none  NoiseParameters=[]  Unit=1  AffineConversion=off  FilteringAndDerivatives=provide  SimscapeFilterOrder=1  InputFilterTimeConstant=0.001  UdotUserProvided=0
  Simulink-PS Converter2 : nesl_utility/Simulink-PS Converter  PhysicalDomain=network_engine_domain  SubClassName=ps_input  LeftPortType=input  RightPortType=output  PseudoPeriodic=off  Frequencies=[]  NoiseDistribution=none  NoiseParameters=[]  Unit=1  AffineConversion=off  FilteringAndDerivatives=provide  SimscapeFilterOrder=1  InputFilterTimeConstant=0.001  UdotUserProvided=0
  Transform Sensor : sm_lib/Frames and Transforms/Transform Sensor  MeasurementFrame=World  SenseAngle=off  SenseAxis=off  SenseQ=off  SenseR=off  SenseRotationSequence=off  RotationSequence=XYX  SenseOmegaX=off  SenseOmegaY=off  SenseOmegaZ=off  SenseQDot=off  SenseRDot=off  SenseAlphaX=off  SenseAlphaY=off  SenseAlphaZ=off  SenseQDDot=off  SenseRDDot=off  SenseX=on  SenseY=on  SenseZ=on  SenseRad=off  SenseAzim=off  SenseDist=off  SenseInc=off  SenseXDot=off  SenseYDot=off  SenseZDot=off  SenseRadDot=off  SenseAzimDot=off  SenseDistDot=off  SenseIncDot=off  SenseXDDot=off  SenseYDDot=off  SenseZDDot=off  SenseRadDDot=off  SenseAzimDDot=off  SenseDistDDot=off  SenseIncDDot=off
  Velocity Concat : Concatenate  NumInputs=3
  Leg Connection : PMIOPort  Side=Left
  Thigh Contact : PMIOPort  Port=2  Side=Left
  Foot Contact : PMIOPort  Port=3  Side=Left
  World Frame : PMIOPort  Port=4  Side=Left
  Angle Vector : Outport
  Velocity Vector : Outport  Port=2
  Foot Pos : Outport  Port=3
  wires:
  torque_vector/1 -> Separate Torques/1(torque_vector)
  Separate Torques/2(thigh_torque) -> Simulink-PS Converter1/1
  Separate Torques/1(hip_torque) -> Simulink-PS Converter/1
  Separate Torques/3(calf_torque) -> Simulink-PS Converter2/1
  Velocity Concat/1 -> Velocity Vector/1
  Angle Concat/1 -> Angle Vector/1
  PS-Simulink Converter4/1 -> Velocity Concat/1
  PS-Simulink Converter3/1 -> Angle Concat/3
  PS-Simulink Converter1/1 -> Angle Concat/1
  PS-Simulink Converter6/1 -> Velocity Concat/3
  PS-Simulink Converter5/1 -> Velocity Concat/2
  PS-Simulink Converter2/1 -> Angle Concat/2
  PS-Simulink Converter9/1 -> Position Concat1/3
  PS-Simulink Converter8/1 -> Position Concat1/2
  PS-Simulink Converter7/1 -> Position Concat1/1
  Position Concat1/1 -> Foot Pos/1
  connections:
  RR_thigh/LConn1 -- RR_thigh_joint/RConn1
  RR_hip/RConn2 -- RR_hip_fixed/LConn1
  RR_hip_joint/LConn1 -- Leg Connection/RConn1
  RR_hip/RConn1 -- RR_thigh_joint/LConn1
  Leg Logger4/LConn3 -- RR_thigh_joint/RConn4
  RR_hip_fixed/RConn1 -- RR_thigh_shoulder/LConn1
  Leg Logger11/LConn3 -- RR_hip_joint/RConn4
  Leg Logger4/LConn2 -- PS-Simulink Converter5/LConn1 -- RR_thigh_joint/RConn3
  RR_calf_joint/RConn3 -- PS-Simulink Converter6/LConn1 -- Leg Logger3/LConn2
  Leg Logger4/LConn1 -- RR_thigh_joint/RConn2 -- PS-Simulink Converter2/LConn1
  Leg Logger11/LConn1 -- PS-Simulink Converter1/LConn1 -- RR_hip_joint/RConn2
  RR_calf_joint/LConn1 -- RR_thigh/RConn2
  Leg Logger11/LConn2 -- PS-Simulink Converter4/LConn1 -- RR_hip_joint/RConn3
  RR_hip/LConn1 -- RR_hip_joint/RConn1
  Thigh Contact/RConn1 -- RR_thigh/RConn1
  Leg Logger3/LConn3 -- RR_calf_joint/RConn4
  RR_calf/RConn1 -- RR_foot_fixed/LConn1
  Leg Logger3/LConn1 -- RR_calf_joint/RConn2 -- PS-Simulink Converter3/LConn1
  RR_calf/LConn1 -- RR_calf_joint/RConn1
  RR_foot_fixed/RConn1 -- Transform Sensor/RConn1 -- RR_foot/LConn1
  RR_foot/LConn2 -- Foot Contact/RConn1
  Simulink-PS Converter1/RConn1 -- RR_thigh_joint/LConn2
  Simulink-PS Converter/RConn1 -- RR_hip_joint/LConn2
  Simulink-PS Converter2/RConn1 -- RR_calf_joint/LConn2
  Transform Sensor/RConn2 -- PS-Simulink Converter7/LConn1
  Transform Sensor/RConn3 -- PS-Simulink Converter8/LConn1
  Transform Sensor/RConn4 -- PS-Simulink Converter9/LConn1
  World Frame/RConn1 -- Transform Sensor/LConn1

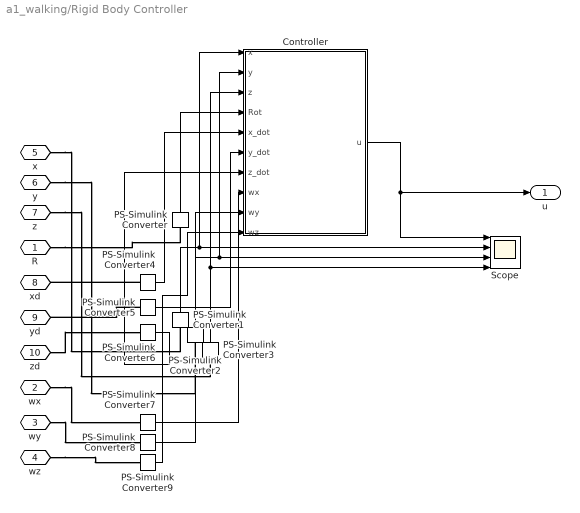
== system a1_walking/Rigid Body Controller ==
  Controller : MATLAB Function  TreatAsAtomicUnit=on
  PS-Simulink Converter{,1..9} (10 alike) : nesl_utility/PS-Simulink Converter  PhysicalDomain=network_engine_domain  SubClassName=ps_output  LeftPortType=input  RightPortType=output  PseudoPeriodic=off  Frequencies=[]  VectorFormat=inherit  Unit=inherit  AffineConversion=off
  Scope : Scope  NumInputPorts=4
  R : PMIOPort  Side=Left
  wx : PMIOPort  Port=2  Side=Left
  wy : PMIOPort  Port=3  Side=Left
  wz : PMIOPort  Port=4  Side=Left
  x : PMIOPort  Port=5  Side=Left
  y : PMIOPort  Port=6  Side=Left
  z : PMIOPort  Port=7  Side=Left
  xd : PMIOPort  Port=8  Side=Left
  yd : PMIOPort  Port=9  Side=Left
  zd : PMIOPort  Port=10  Side=Left
  u : Outport
  wires:
  PS-Simulink Converter2/1 -> Controller/2(y), Scope/3
  PS-Simulink Converter/1 -> Controller/4(Rot)
  Controller/1(u) -> Scope/1, u/1
  PS-Simulink Converter1/1 -> Controller/1(x), Scope/2
  PS-Simulink Converter3/1 -> Controller/3(z), Scope/4
  PS-Simulink Converter4/1 -> Controller/5(x_dot)
  PS-Simulink Converter5/1 -> Controller/6(y_dot)
  PS-Simulink Converter6/1 -> Controller/7(z_dot)
  PS-Simulink Converter7/1 -> Controller/8(wx)
  PS-Simulink Converter8/1 -> Controller/9(wy)
  PS-Simulink Converter9/1 -> Controller/10(wz)
  connections:
  x/RConn1 -- PS-Simulink Converter1/LConn1
  y/RConn1 -- PS-Simulink Converter2/LConn1
  z/RConn1 -- PS-Simulink Converter3/LConn1
  R/RConn1 -- PS-Simulink Converter/LConn1
  PS-Simulink Converter4/LConn1 -- xd/RConn1
  PS-Simulink Converter5/LConn1 -- yd/RConn1
  zd/RConn1 -- PS-Simulink Converter6/LConn1
  wx/RConn1 -- PS-Simulink Converter7/LConn1
  wy/RConn1 -- PS-Simulink Converter8/LConn1
  wz/RConn1 -- PS-Simulink Converter9/LConn1

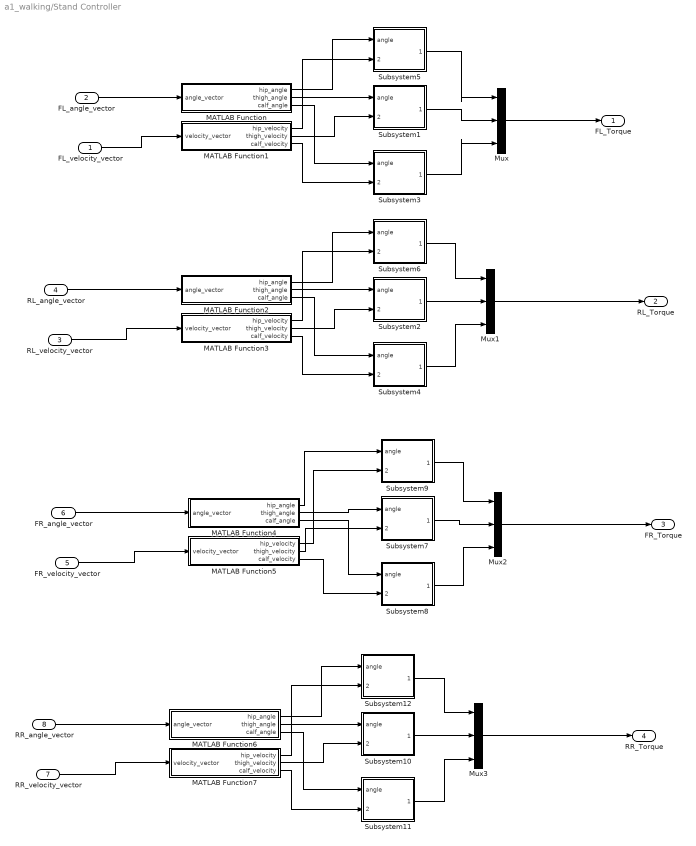
== system a1_walking/Stand Controller ==
  FL_velocity_vector : Inport
  FL_angle_vector : Inport  Port=2
  RL_velocity_vector : Inport  Port=3
  RL_angle_vector : Inport  Port=4
  FR_velocity_vector : Inport  Port=5
  FR_angle_vector : Inport  Port=6
  RR_velocity_vector : Inport  Port=7
  RR_angle_vector : Inport  Port=8
  MATLAB Function : MATLAB Function  TreatAsAtomicUnit=on
  MATLAB Function1 : MATLAB Function  TreatAsAtomicUnit=on
  MATLAB Function2 : MATLAB Function  TreatAsAtomicUnit=on
  MATLAB Function3 : MATLAB Function  TreatAsAtomicUnit=on
  MATLAB Function4 : MATLAB Function  TreatAsAtomicUnit=on
  MATLAB Function5 : MATLAB Function  TreatAsAtomicUnit=on
  MATLAB Function6 : MATLAB Function  TreatAsAtomicUnit=on
  MATLAB Function7 : MATLAB Function  TreatAsAtomicUnit=on
  Mux{,1..3} (4 alike) : Mux  Inputs=3
  Subsystem1 : Subsystem
  Subsystem10 : Subsystem
  Subsystem11 : Subsystem
  Subsystem12 : Subsystem
  Subsystem2 : Subsystem
  Subsystem3 : Subsystem
  Subsystem4 : Subsystem
  Subsystem5 : Subsystem
  Subsystem6 : Subsystem
  Subsystem7 : Subsystem
  Subsystem8 : Subsystem
  Subsystem9 : Subsystem
  FL_Torque : Outport
  RL_Torque : Outport  Port=2
  FR_Torque : Outport  Port=3
  RR_Torque : Outport  Port=4
  wires:
  FL_angle_vector/1 -> MATLAB Function/1(angle_vector)
  MATLAB Function/1(hip_angle) -> Subsystem5/1(angle)
  MATLAB Function1/1(hip_velocity) -> Subsystem5/2(velocity)
  FL_velocity_vector/1 -> MATLAB Function1/1(velocity_vector)
  MATLAB Function/2(thigh_angle) -> Subsystem1/1(angle)
  MATLAB Function1/2(thigh_velocity) -> Subsystem1/2(velocity)
  MATLAB Function/3(calf_angle) -> Subsystem3/1(angle)
  MATLAB Function1/3(calf_velocity) -> Subsystem3/2(velocity)
  Mux/1 -> FL_Torque/1
  Subsystem5/1(Torque) -> Mux/1
  Subsystem1/1(Torque) -> Mux/2
  Subsystem3/1(Torque) -> Mux/3
  RL_angle_vector/1 -> MATLAB Function2/1(angle_vector)
  RL_velocity_vector/1 -> MATLAB Function3/1(velocity_vector)
  MATLAB Function3/1(hip_velocity) -> Subsystem6/2(velocity)
  MATLAB Function2/2(thigh_angle) -> Subsystem2/1(angle)
  MATLAB Function2/1(hip_angle) -> Subsystem6/1(angle)
  MATLAB Function3/3(calf_velocity) -> Subsystem4/2(velocity)
  MATLAB Function3/2(thigh_velocity) -> Subsystem2/2(velocity)
  MATLAB Function2/3(calf_angle) -> Subsystem4/1(angle)
  Mux1/1 -> RL_Torque/1
  Subsystem6/1(Torque) -> Mux1/1
  Subsystem2/1(Torque) -> Mux1/2
  Subsystem4/1(Torque) -> Mux1/3
  FR_velocity_vector/1 -> MATLAB Function5/1(velocity_vector)
  Subsystem7/1(Torque) -> Mux2/2
  MATLAB Function5/2(thigh_velocity) -> Subsystem7/2(velocity)
  Mux2/1 -> FR_Torque/1
  FR_angle_vector/1 -> MATLAB Function4/1(angle_vector)
  Subsystem8/1(Torque) -> Mux2/3
  MATLAB Function4/2(thigh_angle) -> Subsystem7/1(angle)
  Subsystem9/1(Torque) -> Mux2/1
  RR_velocity_vector/1 -> MATLAB Function7/1(velocity_vector)
  MATLAB Function6/3(calf_angle) -> Subsystem11/1(angle)
  MATLAB Function7/1(hip_velocity) -> Subsystem12/2(velocity)
  Subsystem10/1(Torque) -> Mux3/2
  MATLAB Function7/2(thigh_velocity) -> Subsystem10/2(velocity)
  Mux3/1 -> RR_Torque/1
  MATLAB Function7/3(calf_velocity) -> Subsystem11/2(velocity)
  RR_angle_vector/1 -> MATLAB Function6/1(angle_vector)
  Subsystem11/1(Torque) -> Mux3/3
  MATLAB Function6/2(thigh_angle) -> Subsystem10/1(angle)
  Subsystem12/1(Torque) -> Mux3/1
  MATLAB Function6/1(hip_angle) -> Subsystem12/1(angle)
  MATLAB Function4/1(hip_angle) -> Subsystem9/1(angle)
  MATLAB Function5/1(hip_velocity) -> Subsystem9/2(velocity)
  MATLAB Function4/3(calf_angle) -> Subsystem8/1(angle)
  MATLAB Function5/3(calf_velocity) -> Subsystem8/2(velocity)

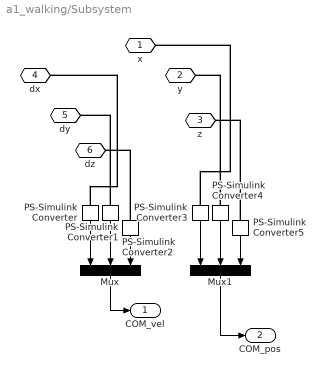
== system a1_walking/Subsystem ==
  Mux : Mux  Inputs=3
  Mux1 : Mux  Inputs=3
  PS-Simulink Converter{,1..5} (6 alike) : nesl_utility/PS-Simulink Converter  PhysicalDomain=network_engine_domain  SubClassName=ps_output  LeftPortType=input  RightPortType=output  PseudoPeriodic=off  Frequencies=[]  VectorFormat=inherit  Unit=inherit  AffineConversion=off
  x : PMIOPort  Side=Left
  y : PMIOPort  Port=2  Side=Left
  z : PMIOPort  Port=3  Side=Left
  dx : PMIOPort  Port=4  Side=Left
  dy : PMIOPort  Port=5  Side=Left
  dz : PMIOPort  Port=6  Side=Left
  COM_vel : Outport
  COM_pos : Outport  Port=2
  wires:
  Mux1/1 -> COM_pos/1
  PS-Simulink Converter2/1 -> Mux/3
  PS-Simulink Converter5/1 -> Mux1/3
  PS-Simulink Converter3/1 -> Mux1/1
  PS-Simulink Converter1/1 -> Mux/2
  Mux/1 -> COM_vel/1
  PS-Simulink Converter4/1 -> Mux1/2
  PS-Simulink Converter/1 -> Mux/1
  connections:
  PS-Simulink Converter3/LConn1 -- x/RConn1
  PS-Simulink Converter2/LConn1 -- dz/RConn1
  PS-Simulink Converter4/LConn1 -- y/RConn1
  PS-Simulink Converter5/LConn1 -- z/RConn1
  PS-Simulink Converter1/LConn1 -- dy/RConn1
  PS-Simulink Converter/LConn1 -- dx/RConn1

== system a1_walking/Swing Controller ==
  COM_velocity : Inport
  t : Inport  Port=2
  T_stance : Inport  Port=3
  v_desired : Inport  Port=4
  MATLAB Function : MATLAB Function  TreatAsAtomicUnit=on
  F : Outport
  wires:
  COM_velocity/1 -> MATLAB Function/1(v_com_vec)
  MATLAB Function/1(F) -> F/1
  t/1 -> MATLAB Function/2(t)
  T_stance/1 -> MATLAB Function/3(T_stance)
  v_desired/1 -> MATLAB Function/4(v_desired)

== system a1_walking/Torque Combiner ==
  In1 : Inport
  Out1 : Outport
  wires:
  In1/1 -> Out1/1

== system a1_walking/Torque Separator ==
  Torque Vector : PMIOPort  Side=Left
  FL Torque Vector : PMIOPort  Port=2  Side=Right
  RL Torque Vector : PMIOPort  Port=3  Side=Right
  FR Torque Vector : PMIOPort  Port=4  Side=Right
  RR Torque Vector : PMIOPort  Port=5  Side=Right

== system a1_walking/Body/Subsystem ==
  Mux1 : Mux  Inputs=3
  PS-Simulink Converter3 : nesl_utility/PS-Simulink Converter  PhysicalDomain=network_engine_domain  SubClassName=ps_output  LeftPortType=input  RightPortType=output  PseudoPeriodic=off  Frequencies=[]  VectorFormat=inherit  Unit=inherit  AffineConversion=off
  PS-Simulink Converter4 : nesl_utility/PS-Simulink Converter  PhysicalDomain=network_engine_domain  SubClassName=ps_output  LeftPortType=input  RightPortType=output  PseudoPeriodic=off  Frequencies=[]  VectorFormat=inherit  Unit=inherit  AffineConversion=off
  PS-Simulink Converter5 : nesl_utility/PS-Simulink Converter  PhysicalDomain=network_engine_domain  SubClassName=ps_output  LeftPortType=input  RightPortType=output  PseudoPeriodic=off  Frequencies=[]  VectorFormat=inherit  Unit=inherit  AffineConversion=off
  x : PMIOPort  Side=Left
  y : PMIOPort  Port=2  Side=Left
  z : PMIOPort  Port=3  Side=Left
  Hip_pos : Outport
  wires:
  Mux1/1 -> Hip_pos/1
  PS-Simulink Converter5/1 -> Mux1/3
  PS-Simulink Converter3/1 -> Mux1/1
  PS-Simulink Converter4/1 -> Mux1/2
  connections:
  PS-Simulink Converter3/LConn1 -- x/RConn1
  PS-Simulink Converter4/LConn1 -- y/RConn1
  PS-Simulink Converter5/LConn1 -- z/RConn1

== system a1_walking/Body/Subsystem1 ==
  Mux1 : Mux  Inputs=3
  PS-Simulink Converter3 : nesl_utility/PS-Simulink Converter  PhysicalDomain=network_engine_domain  SubClassName=ps_output  LeftPortType=input  RightPortType=output  PseudoPeriodic=off  Frequencies=[]  VectorFormat=inherit  Unit=inherit  AffineConversion=off
  PS-Simulink Converter4 : nesl_utility/PS-Simulink Converter  PhysicalDomain=network_engine_domain  SubClassName=ps_output  LeftPortType=input  RightPortType=output  PseudoPeriodic=off  Frequencies=[]  VectorFormat=inherit  Unit=inherit  AffineConversion=off
  PS-Simulink Converter5 : nesl_utility/PS-Simulink Converter  PhysicalDomain=network_engine_domain  SubClassName=ps_output  LeftPortType=input  RightPortType=output  PseudoPeriodic=off  Frequencies=[]  VectorFormat=inherit  Unit=inherit  AffineConversion=off
  x : PMIOPort  Side=Left
  y : PMIOPort  Port=2  Side=Left
  z : PMIOPort  Port=3  Side=Left
  Hip_pos : Outport
  wires:
  Mux1/1 -> Hip_pos/1
  PS-Simulink Converter5/1 -> Mux1/3
  PS-Simulink Converter3/1 -> Mux1/1
  PS-Simulink Converter4/1 -> Mux1/2
  connections:
  PS-Simulink Converter3/LConn1 -- x/RConn1
  PS-Simulink Converter4/LConn1 -- y/RConn1
  PS-Simulink Converter5/LConn1 -- z/RConn1

== system a1_walking/Body/Subsystem2 ==
  Mux1 : Mux  Inputs=3
  PS-Simulink Converter3 : nesl_utility/PS-Simulink Converter  PhysicalDomain=network_engine_domain  SubClassName=ps_output  LeftPortType=input  RightPortType=output  PseudoPeriodic=off  Frequencies=[]  VectorFormat=inherit  Unit=inherit  AffineConversion=off
  PS-Simulink Converter4 : nesl_utility/PS-Simulink Converter  PhysicalDomain=network_engine_domain  SubClassName=ps_output  LeftPortType=input  RightPortType=output  PseudoPeriodic=off  Frequencies=[]  VectorFormat=inherit  Unit=inherit  AffineConversion=off
  PS-Simulink Converter5 : nesl_utility/PS-Simulink Converter  PhysicalDomain=network_engine_domain  SubClassName=ps_output  LeftPortType=input  RightPortType=output  PseudoPeriodic=off  Frequencies=[]  VectorFormat=inherit  Unit=inherit  AffineConversion=off
  x : PMIOPort  Side=Left
  y : PMIOPort  Port=2  Side=Left
  z : PMIOPort  Port=3  Side=Left
  Hip_pos : Outport
  wires:
  Mux1/1 -> Hip_pos/1
  PS-Simulink Converter5/1 -> Mux1/3
  PS-Simulink Converter3/1 -> Mux1/1
  PS-Simulink Converter4/1 -> Mux1/2
  connections:
  PS-Simulink Converter3/LConn1 -- x/RConn1
  PS-Simulink Converter4/LConn1 -- y/RConn1
  PS-Simulink Converter5/LConn1 -- z/RConn1

== system a1_walking/Body/Subsystem3 ==
  Mux1 : Mux  Inputs=3
  PS-Simulink Converter3 : nesl_utility/PS-Simulink Converter  PhysicalDomain=network_engine_domain  SubClassName=ps_output  LeftPortType=input  RightPortType=output  PseudoPeriodic=off  Frequencies=[]  VectorFormat=inherit  Unit=inherit  AffineConversion=off
  PS-Simulink Converter4 : nesl_utility/PS-Simulink Converter  PhysicalDomain=network_engine_domain  SubClassName=ps_output  LeftPortType=input  RightPortType=output  PseudoPeriodic=off  Frequencies=[]  VectorFormat=inherit  Unit=inherit  AffineConversion=off
  PS-Simulink Converter5 : nesl_utility/PS-Simulink Converter  PhysicalDomain=network_engine_domain  SubClassName=ps_output  LeftPortType=input  RightPortType=output  PseudoPeriodic=off  Frequencies=[]  VectorFormat=inherit  Unit=inherit  AffineConversion=off
  x : PMIOPort  Side=Left
  y : PMIOPort  Port=2  Side=Left
  z : PMIOPort  Port=3  Side=Left
  Hip_pos : Outport
  wires:
  Mux1/1 -> Hip_pos/1
  PS-Simulink Converter5/1 -> Mux1/3
  PS-Simulink Converter3/1 -> Mux1/1
  PS-Simulink Converter4/1 -> Mux1/2
  connections:
  PS-Simulink Converter3/LConn1 -- x/RConn1
  PS-Simulink Converter4/LConn1 -- y/RConn1
  PS-Simulink Converter5/LConn1 -- z/RConn1
